simulink model "demo_exakt_siso"  (Simulink 2.20)
settings: Solver=ode45  StartTime=0.0  StopTime=30  MaxStep=0.1  RelTol=1e-3  AbsTol=1e-6
values from neighbouring files (symbols this model uses):
  v = menu('EXACT LINEARIZATION (demo simulations)',    'Exact linearization of SISO system',    'Exact linearization of MIMO system',    'System with unstable zero dynamics')    [demos_exakt.m]    (also in demos_fp.m = menu('PHASE PLANE ANALYSIS (demo simulations)',    '2nd-Orde; demos_gs.m = menu('GAIN SCHEDULING (demo simulations)',    'Input and out)
  x1 = x(j)    [fazrov_auton2.m]
  x2 = x(j+1)    [fazrov_auton2.m]    (also in fazrov_typ1.m = get_param(get_param(gcbh,'Parent'),'UserData'))
libraries: NelinSys x4
settings Model: ConsistencyChecking=off  RTWPlaceOutputsASAP=off

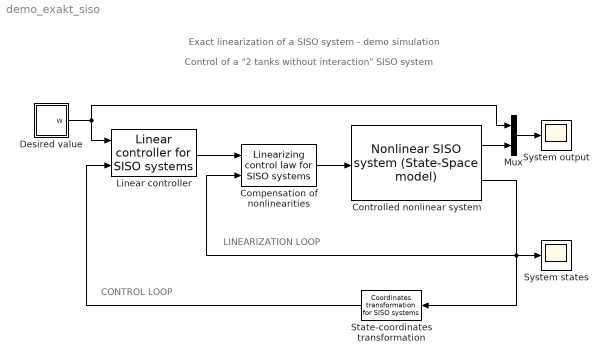
== system demo_exakt_siso ==
  note: LINEARIZATION LOOP
  note: CONTROL LOOP
  note: Exact linearization of a SISO system - demo simulation
  note: Control of a "2 tanks without interaction" SISO system
  Compensation of nonlinearities : NelinSys/Nonlinear Systems Synthesis/Exact Linearization Blocks/Linearizing control law for SISO systems  n=2  vzorec=x1/sqrt(x2)+2*sqrt(x1)*v  vzorecP=0
  Controlled nonlinear system : NelinSys/Nonlinear Systems Synthesis/Nonlinear SISO system (State-Space model)  n=2  F=[-sqrt(x1); sqrt(x1)-sqrt(x2)]  Fp=0  G=[1; 0]  Gp=0  H=x2  Hp=0  pp=[0.1; 0.01]
  "Desired value " : Subsystem
  Linear controller : NelinSys/Nonlinear Systems Synthesis/Exact Linearization Blocks/Linear controller for SISO systems  r=2  kor=[-2 -2]  integ=off
  Mux : Mux  Inputs=2
  State-coordinates transformation : NelinSys/Nonlinear Systems Synthesis/Exact Linearization Blocks/Coordinates transformation for SISO systems  Orientation=left  n=2  r=2  Z=[x2; sqrt(x1)-sqrt(x2)]  Zp=0
  System output : Scope
      settings: TickLabels=on  TimeRange=30  YMin=0  YMax=5  SaveToWorkspace=off  SaveName=ScopeData
  System states : Scope
      settings: TickLabels=on  TimeRange=30  YMin=0  YMax=8  SaveToWorkspace=off  SaveName=ScopeData
  wires:
  Compensation of nonlinearities/1 -> Controlled nonlinear system/1
  Linear controller/1 -> Compensation of nonlinearities/1
  State-coordinates transformation/1 -> Linear controller/2
  Mux/1 -> System output/1
  "Desired value "/1(w) -> Linear controller/1, Mux/1
  Controlled nonlinear system/2 -> State-coordinates transformation/1, Compensation of nonlinearities/2, System states/1
  Controlled nonlinear system/1 -> Mux/2

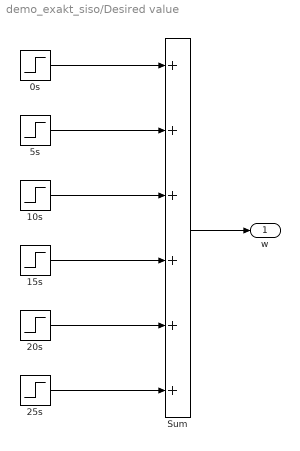
== system demo_exakt_siso/Desired value  ==
  0s : Step  Time=0  Before=0  After=1
  10s : Step  Time=10  Before=0  After=1
  15s : Step  Time=15  Before=0  After=1
  20s : Step  Time=20  Before=0  After=1
  25s : Step  Time=25  Before=0  After=-1
  5s : Step  Time=5  Before=0  After=1
  Sum : Sum  Inputs=++++++
  w : Outport  Port=1
  wires:
  Sum/1 -> w/1
  25s/1 -> Sum/6
  20s/1 -> Sum/5
  15s/1 -> Sum/4
  10s/1 -> Sum/3
  5s/1 -> Sum/2
  0s/1 -> Sum/1
